simulink library "ammclib_bam_S32K11x"  (R2016a)
settings: Solver=VariableStepAuto  SolverMode=SingleTasking  StartTime=0.0  StopTime=10.0  RelTol=1e-3
(part 1 of 16)
settings Model: Creator=ZCZ01vav01-svc  LastModifiedBy=ZCZ01vav01-svc
settings DataIOCC: ReturnWorkspaceOutputs=on
settings DebuggingCC: SFUnexpectedBacktrackingDiag=error  SFNoUnconditionalDefaultTransitionDiag=error
settings SFSimCC: SimUseLocalCustomCode=on
settings RTWCC: RTWUseLocalCustomCode=on
settings GRTTargetCC: TargetLangStandard=C99 (ISO)  GeneratePreprocessorConditionals=Use local settings
settings ConfigComp: CovMetricSettings=dwe  CovHtmlReporting=off  CovSaveCumulativeToWorkspaceVar=off  CovSaveSingleToWorkspaceVar=off  CovExternalEMLEnable=on

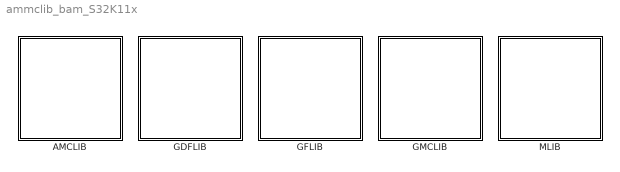
== system ammclib_bam_S32K11x ==
  AMCLIB : Subsystem
  GDFLIB : Subsystem
  GFLIB : Subsystem
  GMCLIB : Subsystem
  MLIB : Subsystem

== system ammclib_bam_S32K11x/AMCLIB ==
  F16 : Subsystem
  F32 : Subsystem

== system ammclib_bam_S32K11x/GDFLIB ==
  F16 : Subsystem
  F32 : Subsystem

== system ammclib_bam_S32K11x/GFLIB ==
  F16 : Subsystem
  F32 : Subsystem

== system ammclib_bam_S32K11x/GMCLIB ==
  F16 : Subsystem
  F32 : Subsystem

== system ammclib_bam_S32K11x/MLIB ==
  F16 : Subsystem
  F32 : Subsystem
  F32F16F16 : Subsystem
